simulink model "02_ee_b"  (R2021a)
settings: Solver=FixedStepDiscrete  StartTime=0.0  StopTime=1  RelTol=1e-3
InitFcn:
  | % Nominal system frequency (Hz)
  |     Fnom= 50;
  | % Number of power module per half-arm
  |     Nb_PM=12;
  | % Nominal DC voltage of one module (V)
  |     Vnom_PM=1000;
  | % Nominal voltage plus DC source
  |     VDCp= (Nb_PM*Vnom_PM)/2;
  | % Nominal voltage minus DC source
  |     VDCm= VDCp;
  | % Initial capacitor DC voltage (V)
  |     Vc_Initial=Vnom_PM;
  | 
  | % Switches parameters:
  | Ron=1e-3;
  | Rs=1e6;
  | Cs=inf;
  | % Power module capacitor (F)
  |     C_PM=5000e-6;
  | % Phase reacter
  |     Lp=20e-3;
  | % SPS Simulation time step(s)
  |     Ts_Power= 10e-6;
  | % Modulator Parameters:
  | % Carriers frequency (Hz)
  |     Fc=Fnom*10;
libraries: spsMultimeterLib x19, spsSeriesRLCBranchLib x11, spsPWMGeneratorMultilevelLib x6, spsHalfBridgeMMCLib x6, spsVoltageMeasurementLib x6, spsGroundLib x2, spsDCVoltageSourceLib x2, spspowerguiLib x1
settings Model: Creator=MathWorks  LastModifiedBy=eagle
settings SolverCC: AlgebraicLoopSolver=TrustRegion
settings DataIOCC: SaveFormat=StructureWithTime  SignalLoggingSaveFormat=ModelDataLogs  SaveOutput=off  SignalLogging=off  DSMLogging=off  SaveTime=off  ReturnWorkspaceOutputs=off
settings OptimizationCC: ExpressionDepthLimit=2147483647  LifeSpan=inf
settings DebuggingCC: UnderspecifiedInitializationDetection=Classic  MergeDetectMultiDrivingBlocksExec=none  SolverPrmCheckMsg=warning  FcnCallInpInsideContextMsg=warning  UnconnectedInputMsg=none  UnconnectedOutputMsg=none  UnconnectedLineMsg=none  AllowSymbolicDim=off  StateNameClashWarn=warning  SFUnexpectedBacktrackingDiag=warning  SFNoUnconditionalDefaultTransitionDiag=warning  SFExecutionAtInitializationDiag=none  SFMachineParentedDataDiag=warning  ArithmeticOperatorsInVariantConditions=warning
settings HardwareCC: ProdBitPerPointer=32  ProdBitPerSizeT=32  ProdBitPerPtrDiffT=32  ProdLargestAtomicFloat=None  ProdIntDivRoundTo=Undefined  ProdEndianess=Unspecified  ProdWordSize=32  ProdHWDeviceType=32-bit Generic
settings ModelReferenceCC: PropagateSignalLabelsOutOfModel=off
settings SFSimCC: SimUseLocalCustomCode=off  CustomCodeUndefinedFunction=UseInterfaceOnly
settings RTWCC: RTWUseLocalCustomCode=off
settings CodeAppCC: StateflowObjectComments=on
settings GRTTargetCC: TargetLangStandard=C89/C90 (ANSI)  CombineOutputUpdateFcns=off  GRTInterface=on
settings ConfigComp: CovMetricSettings=dw  CovSaveCumulativeToWorkspaceVar=on  CovSaveSingleToWorkspaceVar=on  CovExternalEMLEnable=off
settings SimscapeCC: SimscapeNormalizeSystem=off  SimscapeNominalValues={1, 'bar'; 1, 'cm^3/s'; 1, 'bar*kg/s'; 1, 'kJ/kg'; 1, 'kW'; }

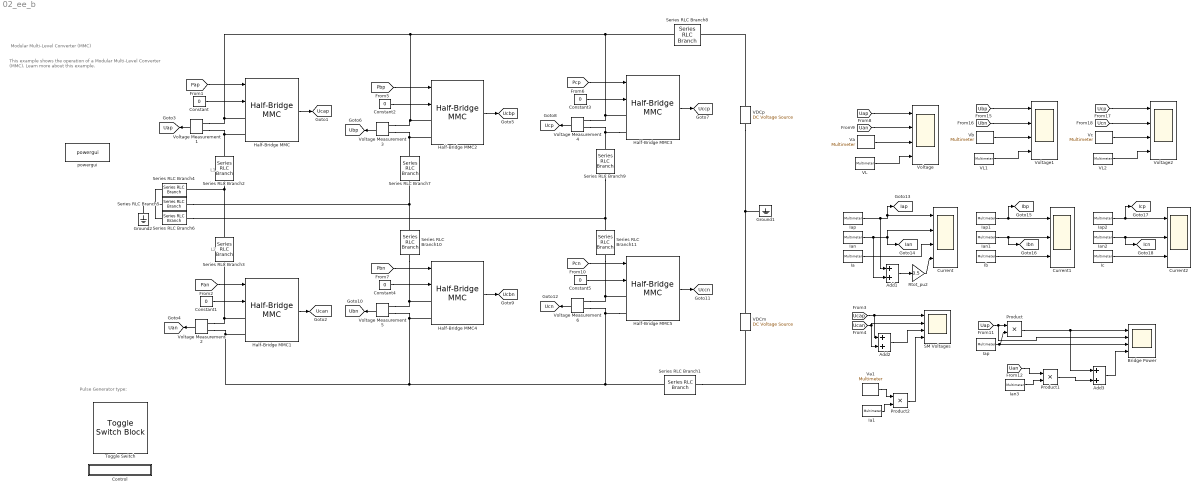
== system 02_ee_b ==
  note: L2
  note: L1
  note: Pulse Generator type:
  note: Modular Multi-Level Converter (MMC)
  note: This example shows the operation of a
      | Modular Multi-Level Converter (MMC).
      |
      | Learn more about this example.
  Add1 : Sum
  Add2 : Sum
  Add3 : Sum
  Bridge Power : Scope  NumInputPorts=4
  Constant{,1..5} (6 alike) : Constant  Value=0
  Control : Subsystem
      mask Display: disp('Control system')
  Current : Scope  NumInputPorts=4
  Current1 : Scope  NumInputPorts=3
  Current2 : Scope  NumInputPorts=3
  Ground1 : spsGroundLib/Ground  LConnTagsString=a
  Ground2 : spsGroundLib/Ground  LConnTagsString=a
  Half-Bridge MMC{,1..5} (6 alike) : spsHalfBridgeMMCLib/Half-Bridge MMC  ModelType=Switching devices  n=Nb_PM  C=C_PM  Vc_Initial=Vc_Initial  Ron=Ron  Rs=Rs  Cs=Cs  Ron_Diode=1e-3  Rs_Diode=1e6  Cs_Diode=inf  Vf_Diode=1e-3  Rs_CurrentSource=inf  Ts=10e-6
      settings: SourceProductBaseCode=PS
  Ia : spsMultimeterLib/Multimeter  PhasorSimulation=off  OutputType=Complex  sel=14  L=18  Gain=1  yselected={'Ib: Series RLC Branch4'};  PSBOutputType=1  PSBequivalent=0  AxesSetting=[0,0.1,-100,100]  Display=0  SavedBlockNames=-11
  Ia1 : spsMultimeterLib/Multimeter  PhasorSimulation=off  OutputType=Complex  sel=14  L=18  Gain=1  yselected={'Ib: Series RLC Branch4'};  PSBOutputType=1  PSBequivalent=0  AxesSetting=[0,0.1,-100,100]  Display=0  SavedBlockNames=-11
  Ian : spsMultimeterLib/Multimeter  PhasorSimulation=off  OutputType=Complex  sel=13  L=18  Gain=1  yselected={'Ib: Series RLC Branch3'};  PSBOutputType=1  PSBequivalent=0  AxesSetting=[0,0.1,-100,100]  Display=0  SavedBlockNames=-11
  Ian1 : spsMultimeterLib/Multimeter  PhasorSimulation=off  OutputType=Complex  sel=10  L=18  Gain=1  yselected={'Ib: Series RLC Branch10'};  PSBOutputType=1  PSBequivalent=0  AxesSetting=[0,0.1,-100,100]  Display=0  SavedBlockNames=-11
  Ian2 : spsMultimeterLib/Multimeter  PhasorSimulation=off  OutputType=Complex  sel=11  L=18  Gain=1  yselected={'Ib: Series RLC Branch11'};  PSBOutputType=1  PSBequivalent=0  AxesSetting=[0,0.1,-100,100]  Display=0  SavedBlockNames=-11
  Ian3 : spsMultimeterLib/Multimeter  PhasorSimulation=off  OutputType=Complex  sel=13  L=18  Gain=1  yselected={'Ib: Series RLC Branch3'};  PSBOutputType=1  PSBequivalent=0  AxesSetting=[0,0.1,-100,100]  Display=0  SavedBlockNames=-11
  Iap : spsMultimeterLib/Multimeter  PhasorSimulation=off  OutputType=Complex  sel=12  L=18  Gain=1  yselected={'Ib: Series RLC Branch2'};  PSBOutputType=1  PSBequivalent=0  AxesSetting=[0,0.1,-100,100]  Display=0  SavedBlockNames=-11
  "Iap " : spsMultimeterLib/Multimeter  PhasorSimulation=off  OutputType=Complex  sel=12  L=18  Gain=1  yselected={'Ib: Series RLC Branch2'};  PSBOutputType=1  PSBequivalent=0  AxesSetting=[0,0.1,-100,100]  Display=0  SavedBlockNames=-11
  Iap1 : spsMultimeterLib/Multimeter  PhasorSimulation=off  OutputType=Complex  sel=17  L=18  Gain=1  yselected={'Ib: Series RLC Branch7'};  PSBOutputType=1  PSBequivalent=0  AxesSetting=[0,0.1,-100,100]  Display=0  SavedBlockNames=-11
  Iap2 : spsMultimeterLib/Multimeter  PhasorSimulation=off  OutputType=Complex  sel=18  L=18  Gain=1  yselected={'Ib: Series RLC Branch9'};  PSBOutputType=1  PSBequivalent=0  AxesSetting=[0,0.1,-100,100]  Display=0  SavedBlockNames=-11
  Ib : spsMultimeterLib/Multimeter  PhasorSimulation=off  OutputType=Complex  sel=6  L=18  Gain=1  yselected={'Ub: Series RLC Branch5'};  PSBOutputType=1  PSBequivalent=0  AxesSetting=[0,0.1,-100,100]  Display=0  SavedBlockNames=-11
  Ic : spsMultimeterLib/Multimeter  PhasorSimulation=off  OutputType=Complex  sel=7  L=18  Gain=1  yselected={'Ub: Series RLC Branch6'};  PSBOutputType=1  PSBequivalent=0  AxesSetting=[0,0.1,-100,100]  Display=0  SavedBlockNames=-11
  Product : Product
  Product1 : Product
  Product2 : Product
  Rtot_pu2 : Gain  Gain=0.5  SaturateOnIntegerOverflow=on  OutDataTypeStr=Inherit: Same as input  ParamDataTypeStr=Inherit: Same as input
  SM Voltages : Scope  NumInputPorts=4
  Series RLC Branch1 : spsSeriesRLCBranchLib/Series RLC Branch  LConnTagsString=__new0  RConnTagsString=__new0  BranchType=RL  Resistance=0.1  Inductance=1e-3  SetiL0=off  InitialCurrent=0  Capacitance=1e-6  Setx0=off  InitialVoltage=0  Measurements=None
  Series RLC Branch{2..3,7,9..11} (6 alike) : spsSeriesRLCBranchLib/Series RLC Branch  LConnTagsString=__new0  RConnTagsString=__new0  BranchType=L  Resistance=1  Inductance=Lp  SetiL0=off  InitialCurrent=0  Capacitance=1e-6  Setx0=off  InitialVoltage=0  Measurements=Branch voltage and current
  Series RLC Branch4 : spsSeriesRLCBranchLib/Series RLC Branch  LConnTagsString=__new0  RConnTagsString=__new0  BranchType=RL  Resistance=50  Inductance=10e-3  SetiL0=off  InitialCurrent=0  Capacitance=1e-6  Setx0=off  InitialVoltage=0  Measurements=Branch voltage and current
  Series RLC Branch5 : spsSeriesRLCBranchLib/Series RLC Branch  LConnTagsString=__new0  RConnTagsString=__new0  BranchType=RL  Resistance=50  Inductance=10e-3  SetiL0=off  InitialCurrent=0  Capacitance=1e-6  Setx0=off  InitialVoltage=0  Measurements=Branch voltage and current
  Series RLC Branch6 : spsSeriesRLCBranchLib/Series RLC Branch  LConnTagsString=__new0  RConnTagsString=__new0  BranchType=RL  Resistance=50  Inductance=10e-3  SetiL0=off  InitialCurrent=0  Capacitance=1e-6  Setx0=off  InitialVoltage=0  Measurements=Branch voltage and current
  Series RLC Branch8 : spsSeriesRLCBranchLib/Series RLC Branch  LConnTagsString=__new0  RConnTagsString=__new0  BranchType=RL  Resistance=0.1  Inductance=1e-3  SetiL0=off  InitialCurrent=0  Capacitance=1e-6  Setx0=off  InitialVoltage=0  Measurements=None
  Toggle Switch : ToggleSwitchBlock  LabelPosition=Hide
      settings: Values={{'Nearest level', 'PWM'}, [0 1]}
  VDCm : spsDCVoltageSourceLib/DC Voltage Source  Amplitude=VDCm  Measurements=None
  VDCp : spsDCVoltageSourceLib/DC Voltage Source  Amplitude=VDCp  Measurements=None
  VL : spsMultimeterLib/Multimeter  PhasorSimulation=off  OutputType=Complex  sel=3  L=18  Gain=1  yselected={'Ub: Series RLC Branch2'};  PSBOutputType=1  PSBequivalent=0  AxesSetting=[0,0.1,-100,100]  Display=0  SavedBlockNames=-11
  VL1 : spsMultimeterLib/Multimeter  PhasorSimulation=off  OutputType=Complex  sel=8  L=18  Gain=1  yselected={'Ub: Series RLC Branch7'};  PSBOutputType=1  PSBequivalent=0  AxesSetting=[0,0.1,-100,100]  Display=0  SavedBlockNames=-11
  VL2 : spsMultimeterLib/Multimeter  PhasorSimulation=off  OutputType=Complex  sel=9  L=18  Gain=1  yselected={'Ub: Series RLC Branch9'};  PSBOutputType=1  PSBequivalent=0  AxesSetting=[0,0.1,-100,100]  Display=0  SavedBlockNames=-11
  Va : spsMultimeterLib/Multimeter  PhasorSimulation=off  OutputType=Complex  sel=5  L=18  Gain=1  yselected={'Ub: Series RLC Branch4'};  PSBOutputType=1  PSBequivalent=0  AxesSetting=[0,0.1,-100,100]  Display=0  SavedBlockNames=-11
  Va1 : spsMultimeterLib/Multimeter  PhasorSimulation=off  OutputType=Complex  sel=5  L=18  Gain=1  yselected={'Ub: Series RLC Branch4'};  PSBOutputType=1  PSBequivalent=0  AxesSetting=[0,0.1,-100,100]  Display=0  SavedBlockNames=-11
  Vb : spsMultimeterLib/Multimeter  PhasorSimulation=off  OutputType=Complex  sel=6  L=18  Gain=1  yselected={'Ub: Series RLC Branch5'};  PSBOutputType=1  PSBequivalent=0  AxesSetting=[0,0.1,-100,100]  Display=0  SavedBlockNames=-11
  Vc : spsMultimeterLib/Multimeter  PhasorSimulation=off  OutputType=Complex  sel=7  L=18  Gain=1  yselected={'Ub: Series RLC Branch6'};  PSBOutputType=1  PSBequivalent=0  AxesSetting=[0,0.1,-100,100]  Display=0  SavedBlockNames=-11
  Voltage : Scope  NumInputPorts=4
  Voltage Measurement{1..6} (6 alike) : spsVoltageMeasurementLib/Voltage Measurement  PhasorSimulation=off  OutputType=Complex  PSBequivalent=0
  Voltage1 : Scope  NumInputPorts=4
  Voltage2 : Scope  NumInputPorts=4
  powergui : spspowerguiLib/powergui  Priority=1  SimulationMode=Discrete  SampleTime=Ts_Power  frequency=60  Iterations=50  frequencyindice=0  Pbase=100e6  ErrMax=1e-4  UnitsV=kV  UnitsW=MW  buscounter=0  FunctionMessages=off  echomessages=off  EnableUseOfTLC=off  CurrentSourceSwitches=off  DisableSnubberDevices=off  DisableRonSwitches=off  DisableVfSwitches=off  DisplayEquations=off  AutomaticDiscreteSolvers=off  SolverType=Tustin/Backward Euler (TBE)  Interpol=off  ExternalGateDelay=off  methode=off  Ts=10  x0status=blocks  SPID=off  SwTol=0  HookPort=off  NonlinearTolerance=1e-4  nMaxIteration=100  ContinueOnMaxIteration=off  RestoreLinks=warning  ResistiveCurrentMeasurement=off  Frange=[0:2:500]  Ylog=off  Xlog=on  ShowGrid=off  save=off  variable=ZData  structure=Vout  ZoomFFT=on  StartTime=0.15  cycles=2  DisplayStyle=1  fundamental=50  FreqAxis=on  MaxFrequency=6000  frequencyindicesteady=1  RmsSteady=1  display=off
  tag scope: Ian=global, Iap=global, Ibn=global, Ibp=global, Icn=global, Icp=global, Uan=global, Uap=global, Ubn=global, Ubp=global, Ucan=global, Ucap=global, Ucbn=global, Ucbp=global, Uccn=global, Uccp=global, Ucn=global, Ucp=global
  wires:
  [Uan] -> Voltage/2
  Va/1 -> Voltage/3
  Iap/1 -> Add1/1, [Iap], Current/1
  Ian/1 -> Add1/2, [Ian], Current/2
  Ia/1 -> Current/3
  VL/1 -> Voltage/4
  [Pap] -> Half-Bridge MMC/1
  Constant/1 -> Half-Bridge MMC/2
  Half-Bridge MMC/1 -> [Ucap]
  Half-Bridge MMC1/1 -> [Ucan]
  Constant1/1 -> Half-Bridge MMC1/2
  [Pan] -> Half-Bridge MMC1/1
  [Uap] -> Voltage/1
  Voltage Measurement1/1 -> [Uap]
  Voltage Measurement2/1 -> [Uan]
  [Ucap] -> Add2/1, SM Voltages/1
  [Ucan] -> Add2/2, SM Voltages/2
  Voltage Measurement3/1 -> [Ubp]
  [Pbp] -> Half-Bridge MMC2/1
  Constant2/1 -> Half-Bridge MMC2/2
  Half-Bridge MMC2/1 -> [Ucbp]
  Voltage Measurement4/1 -> [Ucp]
  [Pcp] -> Half-Bridge MMC3/1
  Constant3/1 -> Half-Bridge MMC3/2
  Half-Bridge MMC3/1 -> [Uccp]
  [Pbn] -> Half-Bridge MMC4/1
  Voltage Measurement5/1 -> [Ubn]
  Half-Bridge MMC4/1 -> [Ucbn]
  Constant4/1 -> Half-Bridge MMC4/2
  Constant5/1 -> Half-Bridge MMC5/2
  [Pcn] -> Half-Bridge MMC5/1
  Voltage Measurement6/1 -> [Ucn]
  Half-Bridge MMC5/1 -> [Uccn]
  Vb/1 -> Voltage1/3
  VL1/1 -> Voltage1/4
  [Ubp] -> Voltage1/1
  [Ubn] -> Voltage1/2
  Vc/1 -> Voltage2/3
  VL2/1 -> Voltage2/4
  [Ucp] -> Voltage2/1
  [Ucn] -> Voltage2/2
  Ib/1 -> Current1/3
  Ian1/1 -> [Ibn], Current1/2
  Iap1/1 -> [Ibp], Current1/1
  Ic/1 -> Current2/3
  Ian2/1 -> [Icn], Current2/2
  Iap2/1 -> [Icp], Current2/1
  Add1/1 -> Rtot_pu2/1
  Rtot_pu2/1 -> Current/4
  Add2/1 -> SM Voltages/3
  [Uap] -> Product/1, Bridge Power/2
  "Iap "/1 -> Bridge Power/3, Product/2
  Product/1 -> Add3/1, Bridge Power/1
  [Uan] -> Product1/1
  Ian3/1 -> Product1/2
  Product1/1 -> Add3/2
  Add3/1 -> Bridge Power/4
  Va1/1 -> Product2/1
  Ia1/1 -> Product2/2
  Product2/1 -> SM Voltages/4
  connections:
  Series RLC Branch2/RConn1 -- Series RLC Branch3/LConn1 -- Series RLC Branch4/LConn1
  Half-Bridge MMC/LConn1 -- Series RLC Branch8/RConn1 -- Voltage Measurement4/LConn1 -- Half-Bridge MMC3/LConn1 -- Half-Bridge MMC2/LConn1 -- Voltage Measurement3/LConn1 -- Voltage Measurement1/LConn1
  Series RLC Branch1/LConn1 -- VDCm/LConn1
  VDCp/LConn1 -- Ground1/LConn1 -- VDCm/RConn1
  Series RLC Branch2/LConn1 -- Voltage Measurement1/LConn2 -- Half-Bridge MMC/LConn2
  Half-Bridge MMC1/LConn1 -- Voltage Measurement2/LConn1 -- Series RLC Branch3/RConn1
  Half-Bridge MMC5/LConn2 -- Series RLC Branch1/RConn1 -- Voltage Measurement5/LConn2 -- Half-Bridge MMC4/LConn2 -- Voltage Measurement2/LConn2 -- Half-Bridge MMC1/LConn2 -- Voltage Measurement6/LConn2
  Series RLC Branch4/RConn1 -- Ground2/LConn1 -- Series RLC Branch5/RConn1 -- Series RLC Branch6/RConn1
  Voltage Measurement3/LConn2 -- Half-Bridge MMC2/LConn2 -- Series RLC Branch7/LConn1
  Half-Bridge MMC3/LConn2 -- Series RLC Branch9/LConn1 -- Voltage Measurement4/LConn2
  Voltage Measurement5/LConn1 -- Series RLC Branch10/RConn1 -- Half-Bridge MMC4/LConn1
  Voltage Measurement6/LConn1 -- Series RLC Branch11/RConn1 -- Half-Bridge MMC5/LConn1
  Series RLC Branch10/LConn1 -- Series RLC Branch5/LConn1 -- Series RLC Branch7/RConn1
  Series RLC Branch9/RConn1 -- Series RLC Branch6/LConn1 -- Series RLC Branch11/LConn1
  VDCp/RConn1 -- Series RLC Branch8/LConn1

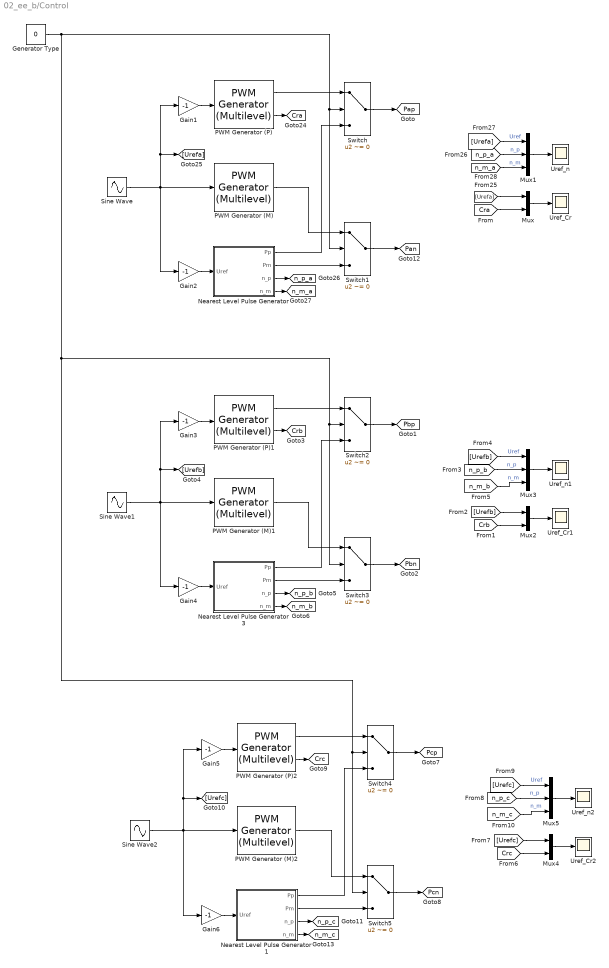
== system 02_ee_b/Control ==
  Gain{1..6} (6 alike) : Gain  Gain=-1
  Generator Type : Constant  Value=0
  Mux : Mux  Inputs=2
  Mux1 : Mux  Inputs=3
  Mux2 : Mux  Inputs=2
  Mux3 : Mux  Inputs=3
  Mux4 : Mux  Inputs=2
  Mux5 : Mux  Inputs=3
  "Nearest Level Pulse Generator " : Subsystem
  Nearest Level Pulse Generator 1 : Subsystem
  Nearest Level Pulse Generator 3 : Subsystem
  PWM Generator (M) : spsPWMGeneratorMultilevelLib/PWM Generator (Multilevel)  BridgeType=Half-bridge  NumberOfBridges=Nb_PM  Fc=Fc  Ts=Ts_Power  ShowCarriersOutport=off
      settings: SourceProductBaseCode=PS
  PWM Generator (M)1 : spsPWMGeneratorMultilevelLib/PWM Generator (Multilevel)  BridgeType=Half-bridge  NumberOfBridges=Nb_PM  Fc=Fc  Ts=Ts_Power  ShowCarriersOutport=off
      settings: SourceProductBaseCode=PS
  PWM Generator (M)2 : spsPWMGeneratorMultilevelLib/PWM Generator (Multilevel)  BridgeType=Half-bridge  NumberOfBridges=Nb_PM  Fc=Fc  Ts=Ts_Power  ShowCarriersOutport=off
      settings: SourceProductBaseCode=PS
  PWM Generator (P) : spsPWMGeneratorMultilevelLib/PWM Generator (Multilevel)  BridgeType=Half-bridge  NumberOfBridges=Nb_PM  Fc=Fc  Ts=Ts_Power  ShowCarriersOutport=on
      settings: SourceProductBaseCode=PS
  PWM Generator (P)1 : spsPWMGeneratorMultilevelLib/PWM Generator (Multilevel)  BridgeType=Half-bridge  NumberOfBridges=Nb_PM  Fc=Fc  Ts=Ts_Power  ShowCarriersOutport=on
      settings: SourceProductBaseCode=PS
  PWM Generator (P)2 : spsPWMGeneratorMultilevelLib/PWM Generator (Multilevel)  BridgeType=Half-bridge  NumberOfBridges=Nb_PM  Fc=Fc  Ts=Ts_Power  ShowCarriersOutport=on
      settings: SourceProductBaseCode=PS
  Sine Wave : Sin  Frequency=2*pi*50  SampleTime=Ts_Power
  Sine Wave1 : Sin  Frequency=2*pi*50  Phase=-2/3*pi  SampleTime=Ts_Power
  Sine Wave2 : Sin  Frequency=2*pi*50  Phase=2/3*pi  SampleTime=Ts_Power
  Switch{,1..5} (6 alike) : Switch  Criteria=u2 ~= 0
  Uref_Cr : Scope
  Uref_Cr1 : Scope
  Uref_Cr2 : Scope
  Uref_n : Scope
  Uref_n1 : Scope
  Uref_n2 : Scope
  tag scope: Cra=global, Crb=global, Crc=global, Pan=global, Pap=global, Pbn=global, Pbp=global, Pcn=global, Pcp=global, n_m_a=global, n_m_b=global, n_m_c=global, n_p_a=global, n_p_b=global, n_p_c=global
  wires:
  Sine Wave/1 -> Gain1/1, [Urefa], PWM Generator (M)/1, Gain2/1
  "Nearest Level Pulse Generator "/1(Pp) -> Switch/3
  PWM Generator (P)/1 -> Switch/1
  Gain1/1 -> PWM Generator (P)/1
  "Nearest Level Pulse Generator "/2(Pm) -> Switch1/3
  Gain2/1 -> "Nearest Level Pulse Generator "/1(Uref)
  Switch/1 -> [Pap]
  PWM Generator (P)/2 -> [Cra]
  Switch1/1 -> [Pan]
  PWM Generator (M)/1 -> Switch1/1
  "Nearest Level Pulse Generator "/3(n_p) -> [n_p_a]
  "Nearest Level Pulse Generator "/4(n_m) -> [n_m_a]
  Mux/1 -> Uref_Cr/1
  [Cra] -> Mux/2
  [Urefa] -> Mux/1
  Mux1/1 -> Uref_n/1
  [n_p_a] -> Mux1/2  "n_p"
  [Urefa] -> Mux1/1  "Uref"
  [n_m_a] -> Mux1/3  "n_m"
  [Urefb] -> Mux2/1
  PWM Generator (M)1/1 -> Switch3/1
  Switch3/1 -> [Pbn]
  Gain4/1 -> Nearest Level Pulse Generator 3/1(Uref)
  [n_m_b] -> Mux3/3  "n_m"
  Mux3/1 -> Uref_n1/1
  Mux2/1 -> Uref_Cr1/1
  [Urefb] -> Mux3/1  "Uref"
  Nearest Level Pulse Generator 3/2(Pm) -> Switch3/3
  [n_p_b] -> Mux3/2  "n_p"
  PWM Generator (P)1/2 -> [Crb]
  [Crb] -> Mux2/2
  Gain3/1 -> PWM Generator (P)1/1
  Nearest Level Pulse Generator 3/1(Pp) -> Switch2/3
  PWM Generator (P)1/1 -> Switch2/1
  Sine Wave1/1 -> Gain3/1, [Urefb], PWM Generator (M)1/1, Gain4/1
  Switch2/1 -> [Pbp]
  Nearest Level Pulse Generator 3/4(n_m) -> [n_m_b]
  Nearest Level Pulse Generator 3/3(n_p) -> [n_p_b]
  Switch4/1 -> [Pcp]
  Mux5/1 -> Uref_n2/1
  Gain6/1 -> Nearest Level Pulse Generator 1/1(Uref)
  Switch5/1 -> [Pcn]
  [Urefc] -> Mux4/1
  PWM Generator (M)2/1 -> Switch5/1
  Nearest Level Pulse Generator 1/3(n_p) -> [n_p_c]
  Nearest Level Pulse Generator 1/4(n_m) -> [n_m_c]
  Sine Wave2/1 -> Gain5/1, [Urefc], PWM Generator (M)2/1, Gain6/1
  [n_m_c] -> Mux5/3  "n_m"
  Nearest Level Pulse Generator 1/2(Pm) -> Switch5/3
  [Urefc] -> Mux5/1  "Uref"
  Mux4/1 -> Uref_Cr2/1
  Generator Type/1 -> Switch5/2, Switch4/2, Switch3/2, Switch2/2, Switch1/2, Switch/2
  Nearest Level Pulse Generator 1/1(Pp) -> Switch4/3
  [Crc] -> Mux4/2
  PWM Generator (P)2/1 -> Switch4/1
  Gain5/1 -> PWM Generator (P)2/1
  PWM Generator (P)2/2 -> [Crc]
  [n_p_c] -> Mux5/2  "n_p"

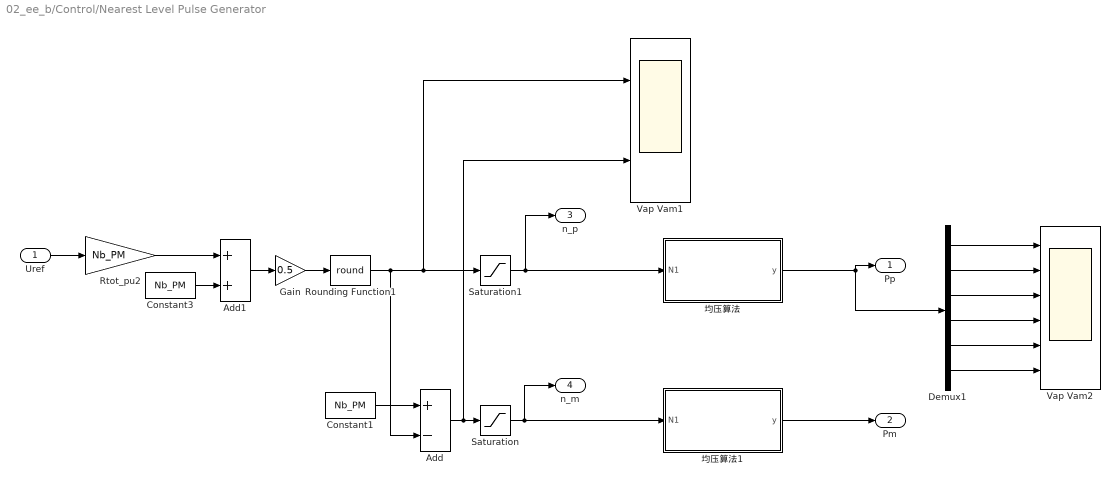
== system 02_ee_b/Control/Nearest Level Pulse Generator  ==
  Uref : Inport
  Add : Sum  Inputs=+-
  Add1 : Sum
  Constant1 : Constant  Value=Nb_PM
  Constant3 : Constant  Value=Nb_PM
  Demux1 : Demux  Outputs=6
  Gain : Gain  Gain=0.5
  Rounding Function1 : Rounding  Operator=round
  Rtot_pu2 : Gain  Gain=Nb_PM  SaturateOnIntegerOverflow=on  OutDataTypeStr=Inherit: Same as input  ParamDataTypeStr=Inherit: Same as input
  Saturation : Saturate  UpperLimit=Nb_PM  LowerLimit=0
  Saturation1 : Saturate  UpperLimit=Nb_PM  LowerLimit=0
  Vap Vam1 : Scope  NumInputPorts=2
  Vap Vam2 : Scope  NumInputPorts=6
  均压算法 : Subsystem
  均压算法1 : Subsystem
  Pp : Outport  VectorParamsAs1DForOutWhenUnconnected=off
  Pm : Outport  Port=2  VectorParamsAs1DForOutWhenUnconnected=off
  n_p : Outport  Port=3  VectorParamsAs1DForOutWhenUnconnected=off
  n_m : Outport  Port=4  VectorParamsAs1DForOutWhenUnconnected=off
  wires:
  Add/1 -> Vap Vam1/2, Saturation/1
  Constant1/1 -> Add/1
  Saturation1/1 -> n_p/1, 均压算法/1(N1)
  Rtot_pu2/1 -> Add1/1
  Constant3/1 -> Add1/2
  Add1/1 -> Gain/1
  Gain/1 -> Rounding Function1/1
  Rounding Function1/1 -> Add/2, Vap Vam1/1, Saturation1/1
  Uref/1 -> Rtot_pu2/1
  Saturation/1 -> n_m/1, 均压算法1/1(N1)
  Demux1/6 -> Vap Vam2/6
  Demux1/3 -> Vap Vam2/3
  Demux1/5 -> Vap Vam2/5
  Demux1/4 -> Vap Vam2/4
  Demux1/1 -> Vap Vam2/1
  Demux1/2 -> Vap Vam2/2
  均压算法/1(y) -> Demux1/1, Pp/1
  均压算法1/1(y) -> Pm/1

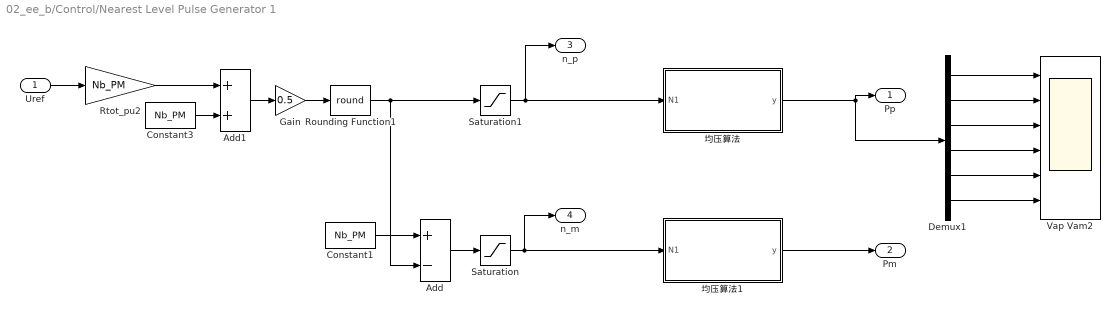
== system 02_ee_b/Control/Nearest Level Pulse Generator 1 ==
  Uref : Inport
  Add : Sum  Inputs=+-
  Add1 : Sum
  Constant1 : Constant  Value=Nb_PM
  Constant3 : Constant  Value=Nb_PM
  Demux1 : Demux  Outputs=6
  Gain : Gain  Gain=0.5
  Rounding Function1 : Rounding  Operator=round
  Rtot_pu2 : Gain  Gain=Nb_PM  SaturateOnIntegerOverflow=on  OutDataTypeStr=Inherit: Same as input  ParamDataTypeStr=Inherit: Same as input
  Saturation : Saturate  UpperLimit=Nb_PM  LowerLimit=0
  Saturation1 : Saturate  UpperLimit=Nb_PM  LowerLimit=0
  Vap Vam2 : Scope  NumInputPorts=6
  均压算法 : Subsystem
  均压算法1 : Subsystem
  Pp : Outport  VectorParamsAs1DForOutWhenUnconnected=off
  Pm : Outport  Port=2  VectorParamsAs1DForOutWhenUnconnected=off
  n_p : Outport  Port=3  VectorParamsAs1DForOutWhenUnconnected=off
  n_m : Outport  Port=4  VectorParamsAs1DForOutWhenUnconnected=off
  wires:
  Add/1 -> Saturation/1
  Constant1/1 -> Add/1
  Saturation1/1 -> n_p/1, 均压算法/1(N1)
  Rtot_pu2/1 -> Add1/1
  Constant3/1 -> Add1/2
  Add1/1 -> Gain/1
  Gain/1 -> Rounding Function1/1
  Rounding Function1/1 -> Add/2, Saturation1/1
  Uref/1 -> Rtot_pu2/1
  Saturation/1 -> n_m/1, 均压算法1/1(N1)
  Demux1/6 -> Vap Vam2/6
  Demux1/3 -> Vap Vam2/3
  Demux1/5 -> Vap Vam2/5
  Demux1/4 -> Vap Vam2/4
  Demux1/1 -> Vap Vam2/1
  Demux1/2 -> Vap Vam2/2
  均压算法/1(y) -> Demux1/1, Pp/1
  均压算法1/1(y) -> Pm/1

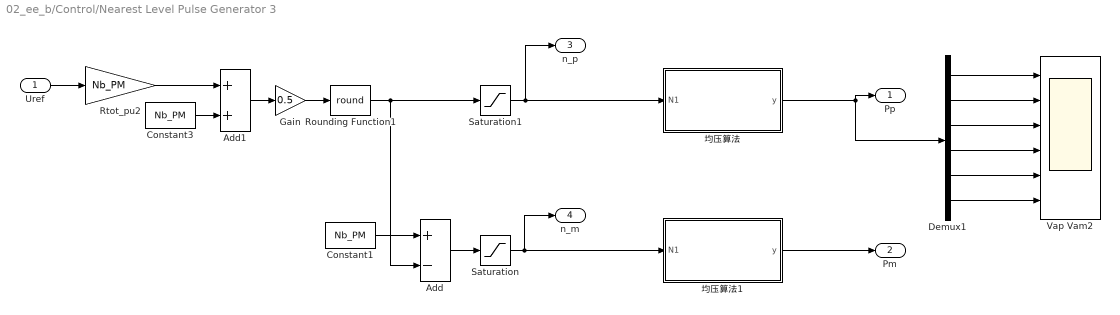
== system 02_ee_b/Control/Nearest Level Pulse Generator 3 ==
  Uref : Inport
  Add : Sum  Inputs=+-
  Add1 : Sum
  Constant1 : Constant  Value=Nb_PM
  Constant3 : Constant  Value=Nb_PM
  Demux1 : Demux  Outputs=6
  Gain : Gain  Gain=0.5
  Rounding Function1 : Rounding  Operator=round
  Rtot_pu2 : Gain  Gain=Nb_PM  SaturateOnIntegerOverflow=on  OutDataTypeStr=Inherit: Same as input  ParamDataTypeStr=Inherit: Same as input
  Saturation : Saturate  UpperLimit=Nb_PM  LowerLimit=0
  Saturation1 : Saturate  UpperLimit=Nb_PM  LowerLimit=0
  Vap Vam2 : Scope  NumInputPorts=6
  均压算法 : Subsystem
  均压算法1 : Subsystem
  Pp : Outport  VectorParamsAs1DForOutWhenUnconnected=off
  Pm : Outport  Port=2  VectorParamsAs1DForOutWhenUnconnected=off
  n_p : Outport  Port=3  VectorParamsAs1DForOutWhenUnconnected=off
  n_m : Outport  Port=4  VectorParamsAs1DForOutWhenUnconnected=off
  wires:
  Add/1 -> Saturation/1
  Constant1/1 -> Add/1
  Saturation1/1 -> n_p/1, 均压算法/1(N1)
  Rtot_pu2/1 -> Add1/1
  Constant3/1 -> Add1/2
  Add1/1 -> Gain/1
  Gain/1 -> Rounding Function1/1
  Rounding Function1/1 -> Add/2, Saturation1/1
  Uref/1 -> Rtot_pu2/1
  Saturation/1 -> n_m/1, 均压算法1/1(N1)
  Demux1/6 -> Vap Vam2/6
  Demux1/3 -> Vap Vam2/3
  Demux1/5 -> Vap Vam2/5
  Demux1/4 -> Vap Vam2/4
  Demux1/1 -> Vap Vam2/1
  Demux1/2 -> Vap Vam2/2
  均压算法/1(y) -> Demux1/1, Pp/1
  均压算法1/1(y) -> Pm/1

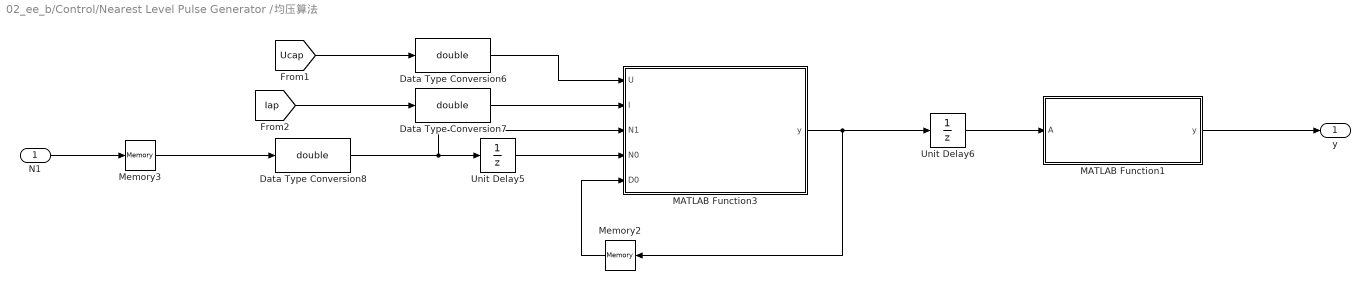
== system 02_ee_b/Control/Nearest Level Pulse Generator /均压算法 ==
  N1 : Inport
  Data Type Conversion6 : DataTypeConversion  OutDataTypeStr=double
  Data Type Conversion7 : DataTypeConversion  OutDataTypeStr=double
  Data Type Conversion8 : DataTypeConversion  OutDataTypeStr=double
  MATLAB Function1 : MATLAB Function  TreatAsAtomicUnit=on
  MATLAB Function3 : MATLAB Function  TreatAsAtomicUnit=on
  Memory2 : Memory
  Memory3 : Memory
  Unit Delay5 : UnitDelay  SampleTime=-1  HasFrameUpgradeWarning=on
  Unit Delay6 : UnitDelay  SampleTime=-1  HasFrameUpgradeWarning=on
  y : Outport
  wires:
  [Ucap] -> Data Type Conversion6/1
  Unit Delay5/1 -> MATLAB Function3/4(N0)
  Data Type Conversion7/1 -> MATLAB Function3/2(I)
  Data Type Conversion6/1 -> MATLAB Function3/1(U)
  Memory2/1 -> MATLAB Function3/5(D0)
  Data Type Conversion8/1 -> MATLAB Function3/3(N1), Unit Delay5/1
  MATLAB Function3/1(y) -> Unit Delay6/1, Memory2/1
  [Iap] -> Data Type Conversion7/1
  Memory3/1 -> Data Type Conversion8/1
  N1/1 -> Memory3/1
  Unit Delay6/1 -> MATLAB Function1/1(A)
  MATLAB Function1/1(y) -> y/1

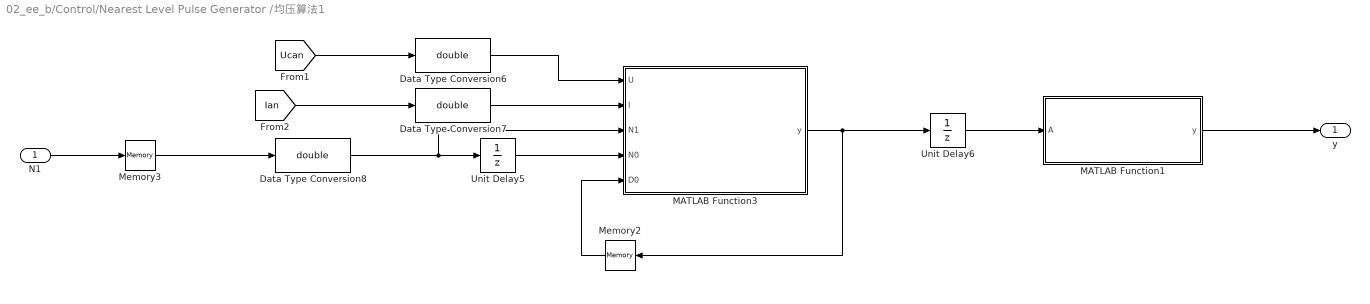
== system 02_ee_b/Control/Nearest Level Pulse Generator /均压算法1 ==
  N1 : Inport
  Data Type Conversion6 : DataTypeConversion  OutDataTypeStr=double
  Data Type Conversion7 : DataTypeConversion  OutDataTypeStr=double
  Data Type Conversion8 : DataTypeConversion  OutDataTypeStr=double
  MATLAB Function1 : MATLAB Function  TreatAsAtomicUnit=on
  MATLAB Function3 : MATLAB Function  TreatAsAtomicUnit=on
  Memory2 : Memory
  Memory3 : Memory
  Unit Delay5 : UnitDelay  SampleTime=-1  HasFrameUpgradeWarning=on
  Unit Delay6 : UnitDelay  SampleTime=-1  HasFrameUpgradeWarning=on
  y : Outport
  wires:
  [Ucan] -> Data Type Conversion6/1
  Unit Delay5/1 -> MATLAB Function3/4(N0)
  Data Type Conversion7/1 -> MATLAB Function3/2(I)
  Data Type Conversion6/1 -> MATLAB Function3/1(U)
  Memory2/1 -> MATLAB Function3/5(D0)
  Data Type Conversion8/1 -> MATLAB Function3/3(N1), Unit Delay5/1
  MATLAB Function3/1(y) -> Unit Delay6/1, Memory2/1
  [Ian] -> Data Type Conversion7/1
  Memory3/1 -> Data Type Conversion8/1
  N1/1 -> Memory3/1
  Unit Delay6/1 -> MATLAB Function1/1(A)
  MATLAB Function1/1(y) -> y/1

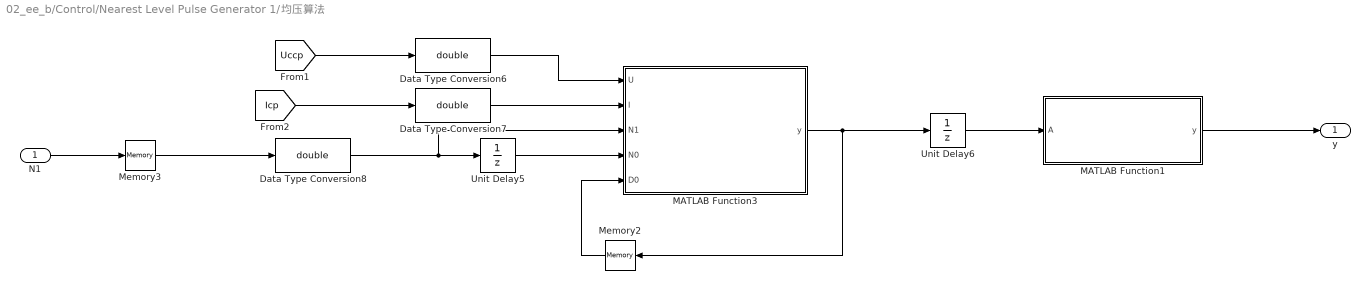
== system 02_ee_b/Control/Nearest Level Pulse Generator 1/均压算法 ==
  N1 : Inport
  Data Type Conversion6 : DataTypeConversion  OutDataTypeStr=double
  Data Type Conversion7 : DataTypeConversion  OutDataTypeStr=double
  Data Type Conversion8 : DataTypeConversion  OutDataTypeStr=double
  MATLAB Function1 : MATLAB Function  TreatAsAtomicUnit=on
  MATLAB Function3 : MATLAB Function  TreatAsAtomicUnit=on
  Memory2 : Memory
  Memory3 : Memory
  Unit Delay5 : UnitDelay  SampleTime=-1  HasFrameUpgradeWarning=on
  Unit Delay6 : UnitDelay  SampleTime=-1  HasFrameUpgradeWarning=on
  y : Outport
  wires:
  [Uccp] -> Data Type Conversion6/1
  Unit Delay5/1 -> MATLAB Function3/4(N0)
  Data Type Conversion7/1 -> MATLAB Function3/2(I)
  Data Type Conversion6/1 -> MATLAB Function3/1(U)
  Memory2/1 -> MATLAB Function3/5(D0)
  Data Type Conversion8/1 -> MATLAB Function3/3(N1), Unit Delay5/1
  MATLAB Function3/1(y) -> Unit Delay6/1, Memory2/1
  [Icp] -> Data Type Conversion7/1
  Memory3/1 -> Data Type Conversion8/1
  N1/1 -> Memory3/1
  Unit Delay6/1 -> MATLAB Function1/1(A)
  MATLAB Function1/1(y) -> y/1

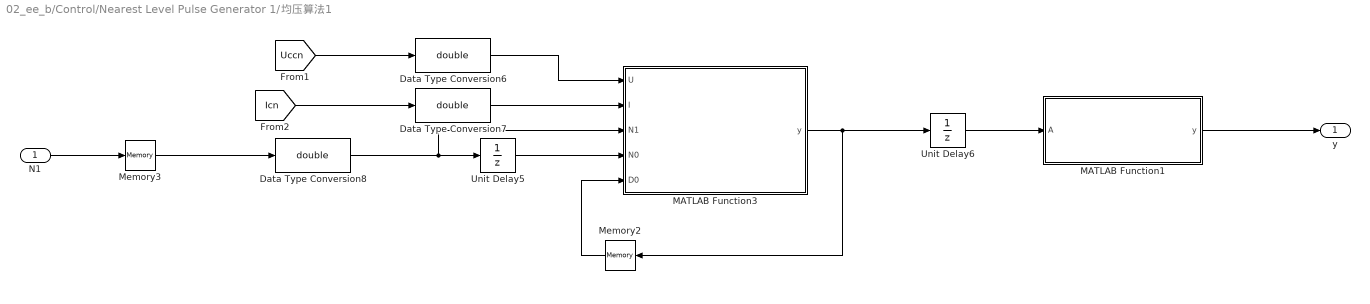
== system 02_ee_b/Control/Nearest Level Pulse Generator 1/均压算法1 ==
  N1 : Inport
  Data Type Conversion6 : DataTypeConversion  OutDataTypeStr=double
  Data Type Conversion7 : DataTypeConversion  OutDataTypeStr=double
  Data Type Conversion8 : DataTypeConversion  OutDataTypeStr=double
  MATLAB Function1 : MATLAB Function  TreatAsAtomicUnit=on
  MATLAB Function3 : MATLAB Function  TreatAsAtomicUnit=on
  Memory2 : Memory
  Memory3 : Memory
  Unit Delay5 : UnitDelay  SampleTime=-1  HasFrameUpgradeWarning=on
  Unit Delay6 : UnitDelay  SampleTime=-1  HasFrameUpgradeWarning=on
  y : Outport
  wires:
  [Uccn] -> Data Type Conversion6/1
  Unit Delay5/1 -> MATLAB Function3/4(N0)
  Data Type Conversion7/1 -> MATLAB Function3/2(I)
  Data Type Conversion6/1 -> MATLAB Function3/1(U)
  Memory2/1 -> MATLAB Function3/5(D0)
  Data Type Conversion8/1 -> MATLAB Function3/3(N1), Unit Delay5/1
  MATLAB Function3/1(y) -> Unit Delay6/1, Memory2/1
  [Icn] -> Data Type Conversion7/1
  Memory3/1 -> Data Type Conversion8/1
  N1/1 -> Memory3/1
  Unit Delay6/1 -> MATLAB Function1/1(A)
  MATLAB Function1/1(y) -> y/1

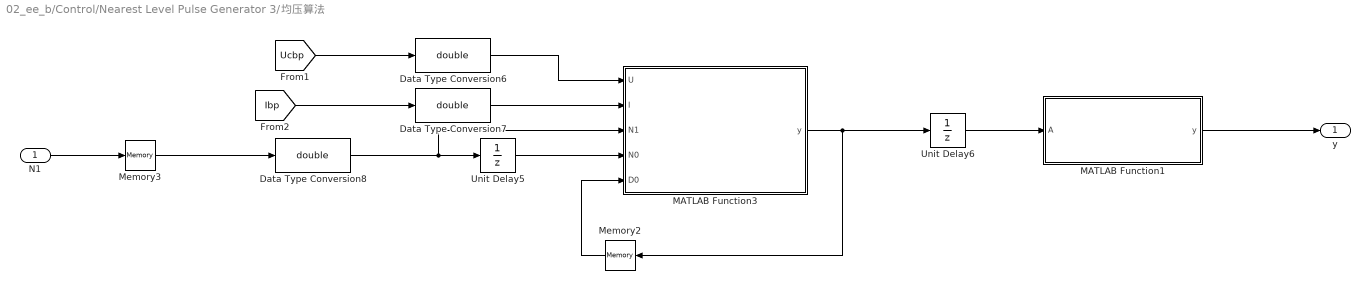
== system 02_ee_b/Control/Nearest Level Pulse Generator 3/均压算法 ==
  N1 : Inport
  Data Type Conversion6 : DataTypeConversion  OutDataTypeStr=double
  Data Type Conversion7 : DataTypeConversion  OutDataTypeStr=double
  Data Type Conversion8 : DataTypeConversion  OutDataTypeStr=double
  MATLAB Function1 : MATLAB Function  TreatAsAtomicUnit=on
  MATLAB Function3 : MATLAB Function  TreatAsAtomicUnit=on
  Memory2 : Memory
  Memory3 : Memory
  Unit Delay5 : UnitDelay  SampleTime=-1  HasFrameUpgradeWarning=on
  Unit Delay6 : UnitDelay  SampleTime=-1  HasFrameUpgradeWarning=on
  y : Outport
  wires:
  [Ucbp] -> Data Type Conversion6/1
  Unit Delay5/1 -> MATLAB Function3/4(N0)
  Data Type Conversion7/1 -> MATLAB Function3/2(I)
  Data Type Conversion6/1 -> MATLAB Function3/1(U)
  Memory2/1 -> MATLAB Function3/5(D0)
  Data Type Conversion8/1 -> MATLAB Function3/3(N1), Unit Delay5/1
  MATLAB Function3/1(y) -> Unit Delay6/1, Memory2/1
  [Ibp] -> Data Type Conversion7/1
  Memory3/1 -> Data Type Conversion8/1
  N1/1 -> Memory3/1
  Unit Delay6/1 -> MATLAB Function1/1(A)
  MATLAB Function1/1(y) -> y/1

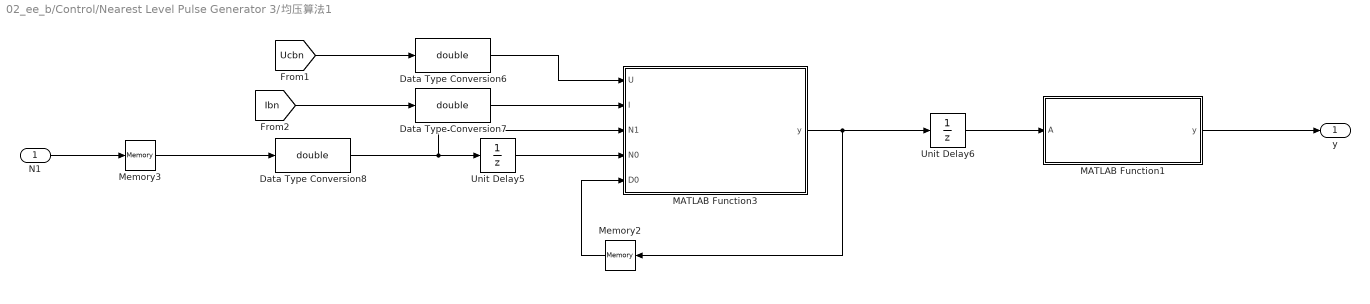
== system 02_ee_b/Control/Nearest Level Pulse Generator 3/均压算法1 ==
  N1 : Inport
  Data Type Conversion6 : DataTypeConversion  OutDataTypeStr=double
  Data Type Conversion7 : DataTypeConversion  OutDataTypeStr=double
  Data Type Conversion8 : DataTypeConversion  OutDataTypeStr=double
  MATLAB Function1 : MATLAB Function  TreatAsAtomicUnit=on
  MATLAB Function3 : MATLAB Function  TreatAsAtomicUnit=on
  Memory2 : Memory
  Memory3 : Memory
  Unit Delay5 : UnitDelay  SampleTime=-1  HasFrameUpgradeWarning=on
  Unit Delay6 : UnitDelay  SampleTime=-1  HasFrameUpgradeWarning=on
  y : Outport
  wires:
  [Ucbn] -> Data Type Conversion6/1
  Unit Delay5/1 -> MATLAB Function3/4(N0)
  Data Type Conversion7/1 -> MATLAB Function3/2(I)
  Data Type Conversion6/1 -> MATLAB Function3/1(U)
  Memory2/1 -> MATLAB Function3/5(D0)
  Data Type Conversion8/1 -> MATLAB Function3/3(N1), Unit Delay5/1
  MATLAB Function3/1(y) -> Unit Delay6/1, Memory2/1
  [Ibn] -> Data Type Conversion7/1
  Memory3/1 -> Data Type Conversion8/1
  N1/1 -> Memory3/1
  Unit Delay6/1 -> MATLAB Function1/1(A)
  MATLAB Function1/1(y) -> y/1

== matlab function 02_ee_b/Control/Nearest Level Pulse Generator /均压算法/MATLAB Function3 ==
  data: U input; y output; I input; N1 input; N0 input; D0 input
function y = Sorting(U,I,N1,N0,D0)
    Np=size(U,1);
    D=zeros(Np,1);%子模块开关状态量 1代表投入 0代表切除

    if N1~=N0    %如果模块数量发生变化，就重新排序 
            
            N=N1;
            
            if  I>0&&N~=0    %电流为正，选择低压模块充电
                [~,B]=sort(U); %B矩阵代表排序后元素在U矩阵的位置
                D(B(1:N))=ones(1,N); %D矩阵在B（i）位置上的值设为1
            end

            if  I<=0&&N~=0  %电流为负，选择高压模块放电电
                [~,B]=sort(U);    
                D(B(Np:-1:(Np-N+1)))=ones(1,N);
            end

            y=D;%输出新的开关量
    else
           y=D0; %模块数量不变，保持输出
    end       
end

== matlab function 02_ee_b/Control/Nearest Level Pulse Generator /均压算法1/MATLAB Function1 ==
  data: A input; y output
function y = IGBT_pulse(A)
[N,~]=size(A);
B=ones(N,1)-A;
C=ones(2*N,1);
for i=1:2*N
    if mod(i,2)==0
        C(i)=B(i/2);
    else
        C(i)=A((i+1)/2);
    end
end
y=C;
end

== matlab function 02_ee_b/Control/Nearest Level Pulse Generator /均压算法1/MATLAB Function3 ==
  data: U input; y output; I input; N1 input; N0 input; D0 input
function y = Sorting(U,I,N1,N0,D0)
    Np=size(U,1);
    D=zeros(Np,1);%子模块开关状态量 1代表投入 0代表切除

    if N1~=N0    %如果模块数量发生变化，就重新排序 
            
            N=N1;
            
            if  I>0&&N~=0    %电流为正，选择低压模块充电
                [~,B]=sort(U); %B矩阵代表排序后元素在U矩阵的位置
                D(B(1:N))=ones(1,N); %D矩阵在B（i）位置上的值设为1
            end

            if  I<=0&&N~=0  %电流为负，选择高压模块放电电
                [~,B]=sort(U);    
                D(B(Np:-1:(Np-N+1)))=ones(1,N);
            end

            y=D;%输出新的开关量
    else
           y=D0; %模块数量不变，保持输出
    end       
end

== matlab function 02_ee_b/Control/Nearest Level Pulse Generator 3/均压算法/MATLAB Function1 ==
  data: A input; y output
function y = IGBT_pulse(A)
[N,~]=size(A);
B=ones(N,1)-A;
C=ones(2*N,1);
for i=1:2*N
    if mod(i,2)==0
        C(i)=B(i/2);
    else
        C(i)=A((i+1)/2);
    end
end
y=C;
end

== matlab function 02_ee_b/Control/Nearest Level Pulse Generator /均压算法/MATLAB Function1 ==
  data: A input; y output
function y = IGBT_pulse(A)
[N,~]=size(A);
B=ones(N,1)-A;
C=ones(2*N,1);
for i=1:2*N
    if mod(i,2)==0
        C(i)=B(i/2);
    else
        C(i)=A((i+1)/2);
    end
end
y=C;
end

== matlab function 02_ee_b/Control/Nearest Level Pulse Generator 3/均压算法/MATLAB Function3 ==
  data: U input; y output; I input; N1 input; N0 input; D0 input
function y = Sorting(U,I,N1,N0,D0)
    Np=size(U,1);
    D=zeros(Np,1);%子模块开关状态量 1代表投入 0代表切除

    if N1~=N0    %如果模块数量发生变化，就重新排序 
            
            N=N1;
            
            if  I>0&&N~=0    %电流为正，选择低压模块充电
                [~,B]=sort(U); %B矩阵代表排序后元素在U矩阵的位置
                D(B(1:N))=ones(1,N); %D矩阵在B（i）位置上的值设为1
            end

            if  I<=0&&N~=0  %电流为负，选择高压模块放电电
                [~,B]=sort(U);    
                D(B(Np:-1:(Np-N+1)))=ones(1,N);
            end

            y=D;%输出新的开关量
    else
           y=D0; %模块数量不变，保持输出
    end       
end

== matlab function 02_ee_b/Control/Nearest Level Pulse Generator 3/均压算法1/MATLAB Function1 ==
  data: A input; y output
function y = IGBT_pulse(A)
[N,~]=size(A);
B=ones(N,1)-A;
C=ones(2*N,1);
for i=1:2*N
    if mod(i,2)==0
        C(i)=B(i/2);
    else
        C(i)=A((i+1)/2);
    end
end
y=C;
end

== matlab function 02_ee_b/Control/Nearest Level Pulse Generator 3/均压算法1/MATLAB Function3 ==
  data: U input; y output; I input; N1 input; N0 input; D0 input
function y = Sorting(U,I,N1,N0,D0)
    Np=size(U,1);
    D=zeros(Np,1);%子模块开关状态量 1代表投入 0代表切除

    if N1~=N0    %如果模块数量发生变化，就重新排序 
            
            N=N1;
            
            if  I>0&&N~=0    %电流为正，选择低压模块充电
                [~,B]=sort(U); %B矩阵代表排序后元素在U矩阵的位置
                D(B(1:N))=ones(1,N); %D矩阵在B（i）位置上的值设为1
            end

            if  I<=0&&N~=0  %电流为负，选择高压模块放电电
                [~,B]=sort(U);    
                D(B(Np:-1:(Np-N+1)))=ones(1,N);
            end

            y=D;%输出新的开关量
    else
           y=D0; %模块数量不变，保持输出
    end       
end

== matlab function 02_ee_b/Control/Nearest Level Pulse Generator 1/均压算法/MATLAB Function1 ==
  data: A input; y output
function y = IGBT_pulse(A)
[N,~]=size(A);
B=ones(N,1)-A;
C=ones(2*N,1);
for i=1:2*N
    if mod(i,2)==0
        C(i)=B(i/2);
    else
        C(i)=A((i+1)/2);
    end
end
y=C;
end

== matlab function 02_ee_b/Control/Nearest Level Pulse Generator 1/均压算法/MATLAB Function3 ==
  data: U input; y output; I input; N1 input; N0 input; D0 input
function y = Sorting(U,I,N1,N0,D0)
    Np=size(U,1);
    D=zeros(Np,1);%子模块开关状态量 1代表投入 0代表切除

    if N1~=N0    %如果模块数量发生变化，就重新排序 
            
            N=N1;
            
            if  I>0&&N~=0    %电流为正，选择低压模块充电
                [~,B]=sort(U); %B矩阵代表排序后元素在U矩阵的位置
                D(B(1:N))=ones(1,N); %D矩阵在B（i）位置上的值设为1
            end

            if  I<=0&&N~=0  %电流为负，选择高压模块放电电
                [~,B]=sort(U);    
                D(B(Np:-1:(Np-N+1)))=ones(1,N);
            end

            y=D;%输出新的开关量
    else
           y=D0; %模块数量不变，保持输出
    end       
end

== matlab function 02_ee_b/Control/Nearest Level Pulse Generator 1/均压算法1/MATLAB Function1 ==
  data: A input; y output
function y = IGBT_pulse(A)
[N,~]=size(A);
B=ones(N,1)-A;
C=ones(2*N,1);
for i=1:2*N
    if mod(i,2)==0
        C(i)=B(i/2);
    else
        C(i)=A((i+1)/2);
    end
end
y=C;
end

== matlab function 02_ee_b/Control/Nearest Level Pulse Generator 1/均压算法1/MATLAB Function3 ==
  data: U input; y output; I input; N1 input; N0 input; D0 input
function y = Sorting(U,I,N1,N0,D0)
    Np=size(U,1);
    D=zeros(Np,1);%子模块开关状态量 1代表投入 0代表切除

    if N1~=N0    %如果模块数量发生变化，就重新排序 
            
            N=N1;
            
            if  I>0&&N~=0    %电流为正，选择低压模块充电
                [~,B]=sort(U); %B矩阵代表排序后元素在U矩阵的位置
                D(B(1:N))=ones(1,N); %D矩阵在B（i）位置上的值设为1
            end

            if  I<=0&&N~=0  %电流为负，选择高压模块放电电
                [~,B]=sort(U);    
                D(B(Np:-1:(Np-N+1)))=ones(1,N);
            end

            y=D;%输出新的开关量
    else
           y=D0; %模块数量不变，保持输出
    end       
end
